simulink model "One_compartment_linear_TOP"  (R2019b)
settings: Solver=VariableStepAuto  StartTime=0.0  StopTime=50  FixedStep=0.01  RelTol=1e-3
values from neighbouring files (symbols this model uses):
  breath = 60/f    (= 4)    [Model_simulation.m]
  E1 = 10    [Model_simulation.m]
  E_high = 100    [Model_simulation.m]
  E_th = 15    [Model_simulation.m]
  insptime = (ieratio(1)/(ieratio(1)+ieratio(2)))*100    [Model_simulation.m]
  Pcontrol = 5    [Model_simulation.m]
  PEEP = 5    [Model_simulation.m]
  R1 = 5    [Model_simulation.m]
  V0 = 2    [Model_simulation.m]
  V0_th = 4.6    [Model_simulation.m]
undefined symbols (not defined in the file or in its folder): TOP
settings Model: Creator=Amne  LastModifiedBy=Amne
settings SolverCC: ZeroCrossAlgorithm=Adaptive  AlgebraicLoopSolver=LineSearch
settings DataIOCC: ReturnWorkspaceOutputsName=SDOSimTest_Log
settings DebuggingCC: IgnoredZcDiagnostic=none  ArithmeticOperatorsInVariantConditions=warning
settings SFSimCC: SimUseLocalCustomCode=off  CustomCodeUndefinedFunction=UseInterfaceOnly
settings RTWCC: RTWUseLocalCustomCode=off

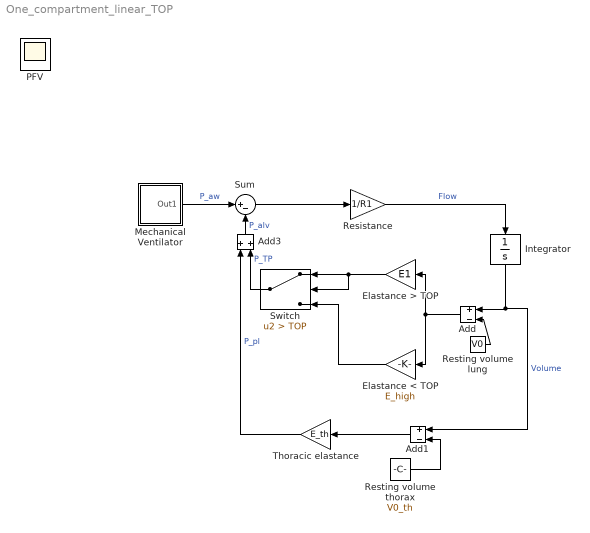
== system One_compartment_linear_TOP ==
  Add : Sum  Inputs=+-
  Add1 : Sum  Inputs=+-
  Add3 : Sum
  Elastance < TOP : Gain  Gain=E_high
  Elastance > TOP : Gain  Gain=E1
  Integrator : Integrator  ZeroCross=off
  "Mechanical Ventilator " : Subsystem
  Resistance : Gain  Gain=1/R1
  Resting volume lung : Constant  Value=V0
  Resting volume thorax : Constant  Value=V0_th
  Sum : Sum  Inputs=|+-
  Switch : Switch  Criteria=u2 > Threshold  Threshold=TOP
  Thoracic elastance : Gain  Gain=E_th
  PFV : Scope
  wires:
  Integrator/1 -> Add1/1, Add/1  "Volume"
  Resistance/1 -> Integrator/1  "Flow"
  Sum/1 -> Resistance/1
  Resting volume lung/1 -> Add/2
  "Mechanical Ventilator "/1(Out1) -> Sum/1  "P_aw"
  Add/1 -> Elastance < TOP/1, Elastance > TOP/1
  Switch/1 -> Add3/2  "P_TP"
  Elastance > TOP/1 -> Switch/2, Switch/1
  Elastance < TOP/1 -> Switch/3
  Resting volume thorax/1 -> Add1/2
  Add1/1 -> Thoracic elastance/1
  Thoracic elastance/1 -> Add3/1  "P_pl"
  Add3/1 -> Sum/2  "P_alv"

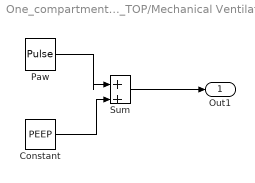
== system One_compartment_linear_TOP/Mechanical Ventilator  ==
  Constant : Constant  Value=PEEP  SampleTime=0.1
  Paw : DiscretePulseGenerator  PulseType=Time based  Amplitude=Pcontrol  Period=breath  PulseWidth=insptime  PhaseDelay=2  SampleTime=0.1
  Sum : Sum  Inputs=|++
  Out1 : Outport  VectorParamsAs1DForOutWhenUnconnected=off
  wires:
  Paw/1 -> Sum/1
  Constant/1 -> Sum/2
  Sum/1 -> Out1/1
